simulink model "UPQC_model"  (R2020b)
settings: Solver=FixedStepAuto  StartTime=0.0  StopTime=Tsim  FixedStep=Tsample  MaxStep=Tsample  RelTol=1e-3
values from neighbouring files (symbols this model uses):
  C_parallel_Series = zeros(1,4)    [Netzmodell_Ini_DL.m]    (also in workspace_Ini.mat = [1e-05 1e-05 1e-05 0])
  C_parallel_Shunt = zeros(1,4)    [Netzmodell_Ini_DL.m]    (also in workspace_Ini.mat = [1e-05 1e-05 1e-05 0])
  CC_Ki = 5    [Netzmodell_Ini_DL.m]    (also in workspace_Ini.mat)
  CC_Ki_geg = 5    [Netzmodell_Ini_DL.m]    (also in workspace_Ini.mat)
  CC_Kp = 10    [Netzmodell_Ini_DL.m]    (also in workspace_Ini.mat)
  CC_Kp_geg = 10    [Netzmodell_Ini_DL.m]    (also in workspace_Ini.mat)
  CC_OS =     [workspace_Ini.mat]
  Czk = Szenario.Czk*u    [Netzmodell_Ini_DL.m]    (also in workspace_Ini.mat = 0.003)
  fak_RVC = Szenario.fak_RVC    [Netzmodell_Ini_DL.m]    (also in workspace_Ini.mat = [1 1 1])
  fak_Uns = [1; 1; 1]    [Netzmodell_Ini_DL.m]    (also in workspace_Ini.mat = [1 1 1])
  Flicker_Schaltzeitpunkte_L1 = Schaltzeitpunkte(1,:)    [Netzmodell_Ini_DL.m]    (also in workspace_Ini.mat = 10.5)
  Flicker_Schaltzeitpunkte_L2 = Schaltzeitpunkte(2,:)    [Netzmodell_Ini_DL.m]    (also in workspace_Ini.mat = 10.5)
  Flicker_Schaltzeitpunkte_L3 = Schaltzeitpunkte(3,:)    [Netzmodell_Ini_DL.m]    (also in workspace_Ini.mat = 10.5)
  fs = [f_nom; f_nom; f_nom]    [Netzmodell_Ini_DL.m]    (also in workspace_Ini.mat = [50 50 50])
  fsw = Szenario.fsw*k    [Netzmodell_Ini_DL.m]    (also in workspace_Ini.mat = 20000)
  I_Basis_Ober_L1 = I_Basis_Ober(1)    [Netzmodell_Ini_DL.m]    (also in workspace_Ini.mat = 0)
  I_Basis_Ober_L2 = I_Basis_Ober(2)    [Netzmodell_Ini_DL.m]    (also in workspace_Ini.mat = 0)
  I_Basis_Ober_L3 = I_Basis_Ober(3)    [Netzmodell_Ini_DL.m]    (also in workspace_Ini.mat = 0)
  I_relativ_Ober_L1 = Szenario.I_relativ_Ober_L1    [Netzmodell_Ini_DL.m]    (also in workspace_Ini.mat = [0 100 0 100 100 0 100 100 0 0 0 0 ... (50 elements, 1x50)])
  I_relativ_Ober_L2 = Szenario.I_relativ_Ober_L2    [Netzmodell_Ini_DL.m]    (also in workspace_Ini.mat = [0 100 0 100 100 0 100 100 0 0 0 0 ... (50 elements, 1x50)])
  I_relativ_Ober_L3 = Szenario.I_relativ_Ober_L3    [Netzmodell_Ini_DL.m]    (also in workspace_Ini.mat = [0 100 0 100 100 0 100 100 0 0 0 0 ... (50 elements, 1x50)])
  L_Ausgang_Series = zeros(1,4)    [Netzmodell_Ini_DL.m]    (also in workspace_Ini.mat = [0.00093 0.00093 0.00093 0.00093])
  L_Ausgang_Shunt = zeros(1,4)    [Netzmodell_Ini_DL.m]    (also in workspace_Ini.mat = [0.00093 0.00093 0.00093 0.00093])
  L_Eingang_Series = zeros(1,4)    [Netzmodell_Ini_DL.m]    (also in workspace_Ini.mat = [0.00085 0.00085 0.00085 0.00085])
  L_Eingang_Shunt = zeros(1,4)    [Netzmodell_Ini_DL.m]    (also in workspace_Ini.mat = [0.00085 0.00085 0.00085 0.00085])
  Ls_in = 52.2*u/10    (= 5.22e-06)    [Netzmodell_Ini_DL.m]    (also in workspace_Ini.mat)
  Ltrans = Szenario.Ltrans*m    [Netzmodell_Ini_DL.m]    (also in workspace_Ini.mat = 0.000256)
  OS_off = 6    [Netzmodell_Ini_DL.m]    (also in workspace_Ini.mat)
  OS_on = 1    [Netzmodell_Ini_DL.m]    (also in workspace_Ini.mat)
  Phi_Ober_L1 = Phi_Ober(1)    [Netzmodell_Ini_DL.m]    (also in workspace_Ini.mat = 0)
  Phi_Ober_L2 = Phi_Ober(2)    [Netzmodell_Ini_DL.m]    (also in workspace_Ini.mat = -120)
  Phi_Ober_L3 = Phi_Ober(3)    [Netzmodell_Ini_DL.m]    (also in workspace_Ini.mat = 120)
  Phis = [0; -120; 120]    [Netzmodell_Ini_DL.m]    (also in workspace_Ini.mat = [0 -120 120])
  Pl_Flicker = Pl_Flicker*k    [Netzmodell_Ini_DL.m]    (also in workspace_Ini.mat = [5000 5000 5000])
  Pl_Grund = Szenario.Pl_Grund *k    [Netzmodell_Ini_DL.m]    (also in workspace_Ini.mat = [5 5 5])
  Pl_RVC = Pl_RVC*k    [Netzmodell_Ini_DL.m]    (also in workspace_Ini.mat = [10000 10000 10000])
  Pl_Uns = Pl_Uns*k    [Netzmodell_Ini_DL.m]    (also in workspace_Ini.mat = [25000 10 10])
  Ql_ind_Flicker = Ql_ind_Flicker*k    [Netzmodell_Ini_DL.m]    (also in workspace_Ini.mat = [0 0 0])
  Ql_ind_Grund = Szenario.Ql_ind_Grund*k    [Netzmodell_Ini_DL.m]    (also in workspace_Ini.mat = [0 0 0])
  Ql_ind_RVC = Szenario.Ql_ind_RVC*k    [Netzmodell_Ini_DL.m]    (also in workspace_Ini.mat = [0 0 0])
  Ql_ind_Uns = Ql_ind_Uns*k    [Netzmodell_Ini_DL.m]    (also in workspace_Ini.mat = [0 0 0])
  Ql_kap_Flicker = Ql_kap_Flicker*k    [Netzmodell_Ini_DL.m]    (also in workspace_Ini.mat = [0 0 0])
  Ql_kap_Grund = Szenario.Ql_kap_Grund*k    [Netzmodell_Ini_DL.m]    (also in workspace_Ini.mat = [0 0 0])
  Ql_kap_RVC = Szenario.Ql_kap_RVC*k    [Netzmodell_Ini_DL.m]    (also in workspace_Ini.mat = [0 0 0])
  Ql_kap_Uns = Ql_kap_Uns*k    [Netzmodell_Ini_DL.m]    (also in workspace_Ini.mat = [0 0 0])
  R_Ausgang_Series = zeros(1,4)    [Netzmodell_Ini_DL.m]    (also in workspace_Ini.mat = [0.1 0.1 0.1 0.1])
  R_Ausgang_Shunt = zeros(1,4)    [Netzmodell_Ini_DL.m]    (also in workspace_Ini.mat = [0.1 0.1 0.1 0.1])
  R_Eingang_Series = zeros(1,4)    [Netzmodell_Ini_DL.m]    (also in workspace_Ini.mat = [0.1 0.1 0.1 0.1])
  R_Eingang_Shunt = zeros(1,4)    [Netzmodell_Ini_DL.m]    (also in workspace_Ini.mat = [0.1 0.1 0.1 0.1])
  R_parallel_Series = zeros(1,4)    [Netzmodell_Ini_DL.m]    (also in workspace_Ini.mat = [13 13 13 0])
  R_parallel_Shunt = zeros(1,4)    [Netzmodell_Ini_DL.m]    (also in workspace_Ini.mat = [13 13 13 0])
  R_ZK_Belastung = 20    [Netzmodell_Ini_DL.m]    (also in workspace_Ini.mat)
  Rs_in = 5.2*m/10    (= 0.00052)    [Netzmodell_Ini_DL.m]    (also in workspace_Ini.mat)
  Rtrans = Szenario.Rtrans    [Netzmodell_Ini_DL.m]    (also in workspace_Ini.mat = 0.206)
  RVC_L1_on_off_Zeitpunkte = Szenario.RVC_L1_on_off_Zeitpunkte    [Netzmodell_Ini_DL.m]    (also in workspace_Ini.mat = [10.5 40 10 11 12 13 14 15])
  RVC_L2_on_off_Zeitpunkte = Szenario.RVC_L2_on_off_Zeitpunkte    [Netzmodell_Ini_DL.m]    (also in workspace_Ini.mat = [10.5 40 10 11 12 13 14 15])
  RVC_L3_on_off_Zeitpunkte = Szenario.RVC_L3_on_off_Zeitpunkte    [Netzmodell_Ini_DL.m]    (also in workspace_Ini.mat = [10.5 40 10 11 12 13 14 15])
  RVC_off = 20.5    [Netzmodell_Ini_DL.m]    (also in workspace_Ini.mat)
  RVC_on = 20    [Netzmodell_Ini_DL.m]    (also in workspace_Ini.mat)
  RVC_val = [0.8,0.8,0.8]    [Netzmodell_Ini_DL.m]    (also in workspace_Ini.mat = [0.8 0.8 0.8])
  strans = Szenario.strans    [Netzmodell_Ini_DL.m]    (also in workspace_Ini.mat = 0.25)
  t_breaker_series = tacts    [Netzmodell_Ini_DL.m]    (also in workspace_Ini.mat = 0.5)
  tact = Szenario.tact    [Netzmodell_Ini_DL.m]    (also in workspace_Ini.mat = 0.5)
  tact_OS_Regler = Szenario.tact_OS_Regler    [Netzmodell_Ini_DL.m]    (also in workspace_Ini.mat = 0.5)
  tact_QU = 10    [Netzmodell_Ini_DL.m]    (also in workspace_Ini.mat)
  tacts = Szenario.tacts    [Netzmodell_Ini_DL.m]    (also in workspace_Ini.mat = 0.5)
  Tsample = Szenario.Tsample    [Netzmodell_Ini_DL.m]    (also in workspace_Ini.mat = 5e-06)
  Uns_L1_on_off_Zeitpunkte = Szenario.Uns_L1_on_off_Zeitpunkte    [Netzmodell_Ini_DL.m]    (also in workspace_Ini.mat = [1 6 10 11 12 13 14 15])
  Uns_L2_on_off_Zeitpunkte = Szenario.Uns_L2_on_off_Zeitpunkte    [Netzmodell_Ini_DL.m]    (also in workspace_Ini.mat = [10 30 10 11 12 13 14 15])
  Uns_L3_on_off_Zeitpunkte = Szenario.Uns_L3_on_off_Zeitpunkte    [Netzmodell_Ini_DL.m]    (also in workspace_Ini.mat = [10 30 10 11 12 13 14 15])
  Us = [Us_Amp; Us_Amp; Us_Amp]    [Netzmodell_Ini_DL.m]    (also in workspace_Ini.mat = [326.598632371 326.598632371 326.598632371])
  Us_Amp = sqrt(2)*400/sqrt(3)    [Netzmodell_Ini_DL.m]    (also in workspace_Ini.mat = 326.598632371)
  VC_Ki_gegen = 30    [Netzmodell_Ini_DL.m]    (also in workspace_Ini.mat)
  VC_Ki_gegen_shunt = 15    [Netzmodell_Ini_DL.m]    (also in workspace_Ini.mat)
  VC_Ki_mit = 5    [Netzmodell_Ini_DL.m]    (also in workspace_Ini.mat)
  VC_Kp_gegen = 5    [workspace_Ini.mat]
  VC_Kp_gegen_shunt = 2    [Netzmodell_Ini_DL.m]    (also in workspace_Ini.mat)
  VC_Kp_mit = 10    [Netzmodell_Ini_DL.m]    (also in workspace_Ini.mat)
  VC_ZK_Ki = 5    [Netzmodell_Ini_DL.m]    (also in workspace_Ini.mat)
  VC_ZK_Kp = 0.5    [Netzmodell_Ini_DL.m]    (also in workspace_Ini.mat)
  Vielfache_Ober_L1 = Szenario.Vielfache_Ober_L1    [Netzmodell_Ini_DL.m]    (also in workspace_Ini.mat = [1 2 3 4 5 6 7 8 9 10 11 12 ... (50 elements, 1x50)])
  Vielfache_Ober_L2 = Szenario.Vielfache_Ober_L2    [Netzmodell_Ini_DL.m]    (also in workspace_Ini.mat = [1 2 3 4 5 6 7 8 9 10 11 12 ... (50 elements, 1x50)])
  Vielfache_Ober_L3 = Szenario.Vielfache_Ober_L3    [Netzmodell_Ini_DL.m]    (also in workspace_Ini.mat = [1 2 3 4 5 6 7 8 9 10 11 12 ... (50 elements, 1x50)])
  ZK_Belastung_off = 100    [Netzmodell_Ini_DL.m]    (also in workspace_Ini.mat)
  ZK_Belastung_on = 100    [Netzmodell_Ini_DL.m]    (also in workspace_Ini.mat)
  Zwischenkreisspannung = 700    [Netzmodell_Ini_DL.m]    (also in workspace_Ini.mat)
undefined symbols (not defined in the file or in its folder): LAusgang, RReiheL3
libraries: powerlib x221, powerlib_meascontrol x80, pid_lib x23, eeTransforms x4, eePwmGeneratorTwoLevel x2, dspstat3 x1
(part 1 of 16)
settings Model: SimulationMode=accelerator  Creator=Emil Weymann  LastModifiedBy=gu92jek
settings SolverCC: ZeroCrossControl=DisableAll  ZeroCrossAlgorithm=Adaptive  AlgebraicLoopSolver=LineSearch
settings DataIOCC: SaveFormat=StructureWithTime  ReturnWorkspaceOutputs=off  LoggingFileName=Messdaten/RVC.mat
settings DebuggingCC: IgnoredZcDiagnostic=none

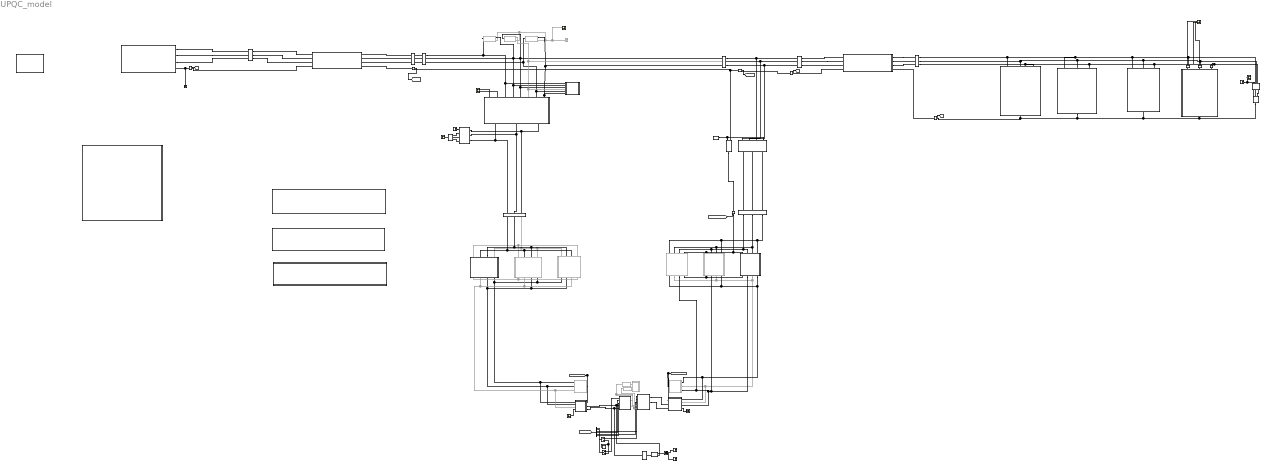
== system UPQC_model ==
  note: Zwischenkreis
  note: Wechselrichter Shunt
  note: Wechselrichter Series
  note: C
  note: (E) Messung Series UPQC
  note: Series Filter UPQC
  note: Shunt Filter UPQC
  note: (D) Messung Shunt UPQC
  note: ON / OFF Series UPQC
  note: (B) Messung UPQC
  note: (C) Messung Last
  note: (A) Messung Ortsnetzstation
  note: Power GUI Block
  note: Leitung
  note: Ortsnetzstation
  note: Lasten
  note: Grundlast
  note: Oberschwingungen Last
  note: Flicker Last
  note: Unsymmetrie Last
  note: RVC Last
  note: ON / OFF Shunt UPQC
  note: B
  note: E
  note: D
  note: A
  note: Messen
  note: Regelung UPQC
  note: Shunt
  note: Series
  note: PLL
  note: Leitung
  note: H
  note: G
  Add : Sum  Inputs=+-
  Breaker Series Control : Step  Commented=on  Time=t_breaker_series  Before=1  SampleTime=0
  Breaker Series Control1 : Step  Time=t_breaker_series  Before=1  After=0  SampleTime=0
  Breaker Shunt Control : powerlib_meascontrol/Pulse & Signal Generators/Stair Generator  t=t_breaker_shunt  e=1  Ts=0
  BreakerCtrlSig_Scope : Scope
  Bus Creator : BusCreator  Inputs=6
  Constant : Constant  Value=700
  Current Measurement{,1..4,6..9} (9 alike) : powerlib/Measurements/Current Measurement  PhasorSimulation=off  OutputType=Complex  PSBequivalent=0
  DC_Quelle_Zwischenkreis : Subsystem  Commented=on  mask{U_Zwischenkreis=Zwischenkreisspannung}
      mask prompts: U_Zwischenkreis "Zwischenkreisspannung [V]"
  Flicker Last : Subsystem  mask{wirk_L1=Pl_Flicker(1), blind_ind_L1=Ql_ind_Flicker(1), blind_kap_L1=Ql_kap_Flicker(1), Schaltzeitpunkte_L1=Flicker_Schaltzeitpunkte_L1, wirk_L2=Pl_Flicker(2), blind_ind_L2=Ql_ind_Flicker(2), blind_kap_L2=Ql_kap_Flicker(2), Schaltzeitpunkte_L2=Flicker_Schaltzeitpunkte_L2, wirk_L3=Pl_Flicker(3), blind_ind_L3=Ql_ind_Flicker(3), blind_kap_L3=Ql_kap_Flicker(3), Schaltzeitpunkte_L3=Flicker_Schaltzeitpunkte_L3}
      mask prompts: wirk_L1 "Wirkleistung[Watt]"; blind_ind_L1 "Blindleistung(Induktiv)[Var]"; blind_kap_L1 "Blindleistung(kapazitiv)[Var]"; Schaltzeitpunkte_L1 "Schaltzeitpunkte"; wirk_L2 "Wirkleistung[Watt]"; blind_ind_L2 "Blindleistung(Induktiv)[Var]"; blind_kap_L2 "Blindleistung(kapazitiv)[Var]"; Schaltzeitpunkte_L2 "Schaltzeitpunkte"; wirk_L3 "Wirkleistung[Watt]"; blind_ind_L3 "Blindleistung(Induktiv)[Var]"; blind_kap_L3 "Blindleistung(kapazitiv)[Var]"; Schaltzeitpunkte_L3 "Schaltzeitpunkte"
      mask DialogControl L1 Prompt: L1
      mask DialogControl L2 Prompt: L2
      mask DialogControl L3 Prompt: L3
  FreilaufDioden_Scope : Scope
  Freilaufdioden : Subsystem
  Ground2 : powerlib/Elements/Ground  LConnTagsString=a
  Grundlast : powerlib/Elements/Three-Phase Parallel RLC Load  LConnTagsString=A|B|C  RConnTagsString=N  Configuration=Y (neutral)  NominalVoltage=1000  Vabc=[400/sqrt(3) 400/sqrt(3) 400/sqrt(3)]  Vabcp=[1e3 1e3 1e3]  NominalFrequency=50  UnbalancedPower=on  ActivePower=10e3  InductivePower=100  CapacitivePower=100  Pabc=[Pl_Grund(1) Pl_Grund(2) Pl_Grund(3)]  QLabc=[Ql_ind_Grund(1) Ql_ind_Grund(2) Ql_ind_Grund(3)]  QCabc=[Ql_kap_Grund(1) Ql_kap_Grund(2) Ql_kap_Grund(3)]  Pabcp=[10e3 9e3 11e3]  QLabcp=[100 90 110]  QCabcp=[100 90 110]  Measurements=None  LoadType=constant PQ
  I_Last_Oberschwingung_Scope : Scope  NumInputPorts=3
  Ideal Switch : powerlib/Power Electronics/Ideal Switch  Ron=0.001  Lon=0  IC=0  Rs=inf  Cs=inf  Measurements=on
  L Filter Series : Subsystem  Commented=on  mask{LEinL1=L_Eingang_Series(1,1), REinL1=R_Eingang_Series(1,1), LEinL2=L_Eingang_Series(1,2), REinL2=R_Eingang_Series(1,2), LEinL3=L_Eingang_Series(1,3), REinL3=R_Eingang_Series(1,3), LEinN=L_Eingang_Series(1,4), REinN=R_Eingang_Series(1,4)}
      mask prompts: LEinL1 "L_Eingang[H]"; REinL1 "R_Eingang[Ohm]"; LEinL2 "L_Eingang[H]"; REinL2 "R_Eingang[Ohm]"; LEinL3 "L_Eingang[H]"; REinL3 "R_Eingang[Ohm]"; LEinN "L_Eingang[H]"; REinN "R_Eingang[Ohm]"
      mask DialogControl ParameterGroupVar Prompt: Parameter für den Filter
      mask DialogControl ContainerL1 Prompt: L1
      mask DialogControl ContainerL2 Prompt: L2
      mask DialogControl ContainerL3 Prompt: L3
      mask DialogControl ContainerN Prompt: N
  L Filter Shunt : Subsystem  Commented=on  mask{LEinL1=L_Eingang_Shunt(1,1), REinL1=R_Eingang_Shunt(1,1), LEinL2=L_Eingang_Shunt(1,2), REinL2=R_Eingang_Shunt(1,2), LEinL3=L_Eingang_Shunt(1,3), REinL3=R_Eingang_Shunt(1,3), LEinN=L_Eingang_Shunt(1,4), REinN=L_Eingang_Shunt(1,4)}
      mask prompts: LEinL1 "L_Eingang[H]"; REinL1 "R_Eingang[Ohm]"; LEinL2 "L_Eingang[H]"; REinL2 "R_Eingang[Ohm]"; LEinL3 "L_Eingang[H]"; REinL3 "R_Eingang[Ohm]"; LEinN "L_Eingang[H]"; REinN "R_Eingang[Ohm]"
      mask DialogControl ParameterGroupVar Prompt: Parameter für den Filter
      mask DialogControl ContainerL1 Prompt: L1
      mask DialogControl ContainerL2 Prompt: L2
      mask DialogControl ContainerL3 Prompt: L3
      mask DialogControl ContainerN Prompt: N
  L1 Breaker Series : powerlib/Elements/Breaker  Commented=on  InitialState=1  SwitchingTimes="[1/60  5/60]"  External=on  BreakerResistance=0.01  SnubberResistance=1e6  SnubberCapacitance=inf  Measurements=None  MoreParameters=on  NoBreakLoop=off
  L2 Breaker Series : powerlib/Elements/Breaker  Commented=on  InitialState=1  SwitchingTimes="[1/60  5/60]"  External=on  BreakerResistance=0.01  SnubberResistance=1e6  SnubberCapacitance=inf  Measurements=None  MoreParameters=on  NoBreakLoop=off
  L3 Breaker Series : powerlib/Elements/Breaker  Commented=on  InitialState=1  SwitchingTimes="[1/60  5/60]"  External=on  BreakerResistance=0.01  SnubberResistance=1e6  SnubberCapacitance=inf  Measurements=None  MoreParameters=on  NoBreakLoop=off
  LC Filter Series : Subsystem  Commented=on  mask{LEinL1=L_Eingang_Series(1,1)*3, CL1=C_parallel_Series(1,1)*750, REinL1=R_Eingang_Series(1,1), RReiheL1=R_parallel_Series(1,1), LEinL2=L_Eingang_Series(1,2)*3, CL2=C_parallel_Series(1,2)*750, REinL2=R_Eingang_Series(1,2), RReiheL2=R_parallel_Series(1,2), LEinL3=L_Eingang_Series(1,3)*3, CL3=C_parallel_Series(1,3)*750, REinL3=R_Eingang_Series(1,3), RReiheL3=R_parallel_Series(1,3), LEinN=L_Eingang_Series(1,4), REinN=R_Eingang_Series(1,4)}
      mask prompts: LEinL1 "L_Eingang[H]"; CL1 "C[F]"; REinL1 "R_Eingang[Ohm]"; RReiheL1 "R in Reihe C[Ohm]"; LEinL2 "L_Eingang[H]"; CL2 "C[F]"; REinL2 "R_Eingang[Ohm]"; RReiheL2 "R in Reihe C[Ohm]"; LEinL3 "L_Eingang[H]"; CL3 "C[F]"; REinL3 "R_Eingang[Ohm]"; RReiheL3 "R in Reihe C[Ohm]"; LEinN "L_Eingang[H]"; REinN "R_Eingang[Ohm]"
      mask DialogControl ParameterGroupVar Prompt: Parameter für den Filter
      mask DialogControl ContainerL1 Prompt: L1
      mask DialogControl ContainerL2 Prompt: L2
      mask DialogControl ContainerL3 Prompt: L3
      mask DialogControl ContainerN Prompt: N
  LC Filter Shunt : Subsystem  Commented=on  mask{LEinL1=L_Eingang_Shunt(1,1), CL1=C_parallel_Shunt(1,1), REinL1=R_Eingang_Shunt(1,1), RReiheL1=R_parallel_Shunt(1,1), LEinL2=L_Eingang_Shunt(1,2), CL2=C_parallel_Shunt(1,2), REinL2=R_Eingang_Shunt(1,2), RReiheL2=R_parallel_Shunt(1,2), LEinL3=L_Eingang_Shunt(1,3), CL3=C_parallel_Shunt(1,3), REinL3=R_Eingang_Shunt(1,3), RReiheL3=R_parallel_Shunt(1,3), LEinN=0, REinN=0}
      mask prompts: LEinL1 "L_Eingang[H]"; CL1 "C[F]"; REinL1 "R_Eingang[Ohm]"; RReiheL1 "R in Reihe C[Ohm]"; LEinL2 "L_Eingang[H]"; CL2 "C[F]"; REinL2 "R_Eingang[Ohm]"; RReiheL2 "R in Reihe C[Ohm]"; LEinL3 "L_Eingang[H]"; CL3 "C[F]"; REinL3 "R_Eingang[Ohm]"; RReiheL3 "R in Reihe C[Ohm]"; LEinN "L_Eingang[H]"; REinN "R_Eingang[Ohm]"
      mask DialogControl ParameterGroupVar Prompt: Parameter für den Filter
      mask DialogControl ContainerL1 Prompt: L1
      mask DialogControl ContainerL2 Prompt: L2
      mask DialogControl ContainerL3 Prompt: L3
      mask DialogControl ContainerN Prompt: N
  LCL Filter Series : Subsystem  mask{LEinL1=L_Eingang_Series(1,1), LAusL1=L_Ausgang_Series(1,1), CL1=C_parallel_Series(1,1), REinL1=R_Eingang_Series(1,1), RAusL1=R_Ausgang_Series(1,1), RReiheL1=R_parallel_Series(1,1), LEinL2=L_Eingang_Series(1,2), LAusL2=L_Ausgang_Series(1,2), CL2=C_parallel_Series(1,2), REinL2=R_Eingang_Series(1,2), RAusL2=R_Ausgang_Series(1,2), RReiheL2=R_parallel_Series(1,2), LEinL3=L_Eingang_Series(1,3), LAusL3=L_Ausgang_Series(1,3), CL3=C_parallel_Series(1,3), REinL3=R_Eingang_Series(1,3), RAusL3=R_Ausgang_Series(1,3), RReiheL3=R_parallel_Series(1,3), LEinN=L_Eingang_Series(1,4), LAusN=L_Ausgang_Series(1,4), REinN=R_Eingang_Series(1,4), RAusN=R_Ausgang_Series(1,4)}
      mask prompts: LEinL1 "L_Eingang[H]"; LAusL1 "L_Ausgang[H]"; CL1 "C[F]"; REinL1 "R_Eingang[Ohm]"; RAusL1 "R_Ausgang[Ohm]"; RReiheL1 "R in Reihe C[Ohm]"; LEinL2 "L_Eingang[H]"; LAusL2 "L_Ausgang[H]"; CL2 "C[F]"; REinL2 "R_Eingang[Ohm]"; RAusL2 "R_Ausgang[Ohm]"; RReiheL2 "R in Reihe C[Ohm]"; LEinL3 "L_Eingang[H]"; LAusL3 "L_Ausgang[H]"; CL3 "C[F]"; REinL3 "R_Eingang[Ohm]"; RAusL3 "R_Ausgang[Ohm]"; RReiheL3 "R in Reihe C[Ohm]"; LEinN "L_Eingang[H]"; LAusN "L_Ausgang[H]"; REinN "R_Eingang[Ohm]"; RAusN "R_Ausgang[Ohm]"
      mask DialogControl ParameterGroupVar Prompt: Parameter für den Filter
      mask DialogControl ContainerL1 Prompt: L1
      mask DialogControl ContainerL2 Prompt: L2
      mask DialogControl ContainerL3 Prompt: L3
      mask DialogControl ContainerN Prompt: N
  LCL Filter Shunt : Subsystem  mask{LEinL1=L_Eingang_Shunt(1,1), LAusL1=L_Ausgang_Shunt(1,1), CL1=C_parallel_Shunt(1,1), REinL1=R_Eingang_Shunt(1,1), RAusL1=R_Ausgang_Shunt(1,1), RReiheL1=R_parallel_Shunt(1,1), LEinL2=L_Eingang_Shunt(1,2), LAusL2=L_Ausgang_Shunt(1,2), CL2=C_parallel_Shunt(1,2), REinL2=R_Eingang_Shunt(1,2), RAusL2=R_Ausgang_Shunt(1,2), RReiheL2=R_parallel_Shunt(1,2), LEinL3=L_Eingang_Shunt(1,3), LAusL3=L_Ausgang_Shunt(1,3), CL3=C_parallel_Shunt(1,3), REinL3=R_Eingang_Shunt(1,3), RAusL3=R_Ausgang_Shunt(1,3), RReiheL3=R_parallel_Shunt(1,3), LEinN=L_Eingang_Shunt(1,4), LAusN=L_Ausgang_Shunt(1,4), REinN=R_Eingang_Shunt(1,4), RAusN=R_Ausgang_Shunt(1,4)}
      mask prompts: LEinL1 "L_Eingang[H]"; LAusL1 "L_Ausgang[H]"; CL1 "C[F]"; REinL1 "R_Eingang[Ohm]"; RAusL1 "R_Ausgang[Ohm]"; RReiheL1 "R in Reihe C[Ohm]"; LEinL2 "L_Eingang[H]"; LAusL2 "L_Ausgang[H]"; CL2 "C[F]"; REinL2 "R_Eingang[Ohm]"; RAusL2 "R_Ausgang[Ohm]"; RReiheL2 "R in Reihe C[Ohm]"; LEinL3 "L_Eingang[H]"; LAusL3 "L_Ausgang[H]"; CL3 "C[F]"; REinL3 "R_Eingang[Ohm]"; RAusL3 "R_Ausgang[Ohm]"; RReiheL3 "R in Reihe C[Ohm]"; LEinN "L_Eingang[H]"; LAusN "L_Ausgang[H]"; REinN "R_Eingang[Ohm]"; RAusN "R_Ausgang[Ohm]"
      mask DialogControl ParameterGroupVar Prompt: Parameter für den Filter
      mask DialogControl ContainerL1 Prompt: L1
      mask DialogControl ContainerL2 Prompt: L2
      mask DialogControl ContainerL3 Prompt: L3
      mask DialogControl ContainerN Prompt: N
  Leitungsnachbildung RL : Subsystem  mask{R_pro_KM=Rtrans, L_pro_KM=Ltrans, KM=strans}
      mask prompts: R_pro_KM "Widerstandsbelag(Ohm_pro_KM)"; L_pro_KM "Induktivitätsbelag(H_pro_KM)"; KM "Länge(Km)"
  Leitungsnachbildung RL1 : Subsystem  mask{R_pro_KM=Rtrans, L_pro_KM=Ltrans, KM=strans}
      mask prompts: R_pro_KM "Widerstandsbelag(Ohm_pro_KM)"; L_pro_KM "Induktivitätsbelag(H_pro_KM)"; KM "Länge(Km)"
  Manual Switch : ManualSwitch
  Manual Switch1 : ManualSwitch
  Measurement Transformer : Subsystem
  Messpunkt C : powerlib/Measurements/Three-Phase V-I Measurement  VoltageMeasurement=phase-to-ground  SetLabelV=on  LabelV=Vabc_C  Vpu=off  VpuLL=off  CurrentMeasurement=yes  SetLabelI=on  LabelI=Iabc_C  Ipu=off  Pbase=100e6  Vbase=500e3  OutputType=Complex  PhasorSimulation=off  PSBequivalent=0
  Messpunkt G : powerlib/Measurements/Three-Phase V-I Measurement  VoltageMeasurement=phase-to-ground  SetLabelV=on  LabelV=Vabc_G  Vpu=off  VpuLL=off  CurrentMeasurement=yes  SetLabelI=on  LabelI=Iabc_G  Ipu=off  Pbase=100e6  Vbase=500e3  OutputType=Complex  PhasorSimulation=off  PSBequivalent=0
  Messpunkt H : powerlib/Measurements/Three-Phase V-I Measurement  VoltageMeasurement=phase-to-ground  SetLabelV=on  LabelV=Vabc_H  Vpu=off  VpuLL=off  CurrentMeasurement=yes  SetLabelI=on  LabelI=Iabc_H  Ipu=off  Pbase=100e6  Vbase=500e3  OutputType=Complex  PhasorSimulation=off  PSBequivalent=0
  Messsignale : Subsystem
  N Breaker Shunt : powerlib/Elements/Breaker  InitialState=0  SwitchingTimes="[1/60  5/60]"  External=on  BreakerResistance=0.01  SnubberResistance=1e6  SnubberCapacitance=inf  Measurements=None  MoreParameters=on  NoBreakLoop=off
  Oberschwingung Last : Subsystem  mask{amp_L1=I_relativ_Ober_L1, BasisStromL1=I_Basis_Ober_L1, O_L1=Vielfache_Ober_L1, phase_L1=Phi_Ober_L1, init_amp_L1=0, init_phase_L1=0, init_freq_L1=50, amp_L2=I_relativ_Ober_L2, BasisStromL2=I_Basis_Ober_L2, O_L2=Vielfache_Ober_L2, phase_L2=Phi_Ober_L2, init_amp_L2=0, init_phase_L2=0, init_freq_L2=50, amp_L3=I_relativ_Ober_L3, BasisStromL3=I_Basis_Ober_L3, O_L3=Vielfache_Ober_L3, phase_L3=Phi_Ober_L3, init_amp_L3=0, init_phase_L3=0, init_freq_L3=50}
      mask prompts: amp_L1 "Amplitude von Basistrom(50Hz)[%] (Dimension n)"; BasisStromL1 "Basisstrom (bei 50Hz oder 1.Harmonische) [A] (Dimension 1)"; O_L1 "Vielfache von 50 Hz (Dimension n)"; phase_L1 "Phase[Grad] (Dimension 1)"; init_amp_L1 "Initial_Amplitude[A] (Dimension 1)"; init_phase_L1 "Initial_Phase[Grad] (Dimension 1)"; init_freq_L1 "Initial_Frequenz[Hz] (Dimension 1)"; amp_L2 "Amplitude von Basistrom(50Hz)[%] (Dimension n)"; BasisStromL2 "Basisstrom (bei 50Hz oder 1.Harmonische) [A] (Dimension 1)"; O_L2 "Vielfache von 50 Hz (Dimension n)"; phase_L2 "Phase[Grad] (Dimension 1)"; init_amp_L2 "Initial_Amplitude[A] (Dimension 1)"; init_phase_L2 "Initial_Phase[Grad] (Dimension 1)"; init_freq_L2 "Initial_Frequenz[Hz] (Dimension 1)"; amp_L3 "Amplitude von Basistrom(50Hz)[%] (Dimension n)"; BasisStromL3 "Basisstrom (bei 50Hz oder 1.Harmonische) [A] (Dimension 1)"; O_L3 "Vielfache von 50 Hz (Dimension n)"; phase_L3 "Phase[Grad] (Dimension 1)"; init_amp_L3 "Initial_Amplitude[A] (Dimension 1)"; init_phase_L3 "Initial_Phase[Grad] (Dimension 1)"; init_freq_L3 "Initial_Frequenz[Hz] (Dimension 1)"
      mask DialogControl L1 Prompt: L1
      mask DialogControl L2 Prompt: L2
      mask DialogControl L3 Prompt: L3
  Position 1 : powerlib/Measurements/Three-Phase V-I Measurement  VoltageMeasurement=phase-to-ground  SetLabelV=on  LabelV=Vabc_A  Vpu=off  VpuLL=off  CurrentMeasurement=yes  SetLabelI=on  LabelI=Iabc_A  Ipu=off  Pbase=100e6  Vbase=500e3  OutputType=Complex  PhasorSimulation=off  PSBequivalent=0
  Position 2 : powerlib/Measurements/Three-Phase V-I Measurement  VoltageMeasurement=phase-to-ground  SetLabelV=on  LabelV=Vabc_B  Vpu=off  VpuLL=off  CurrentMeasurement=yes  SetLabelI=on  LabelI=Iabc_B  Ipu=off  Pbase=100e6  Vbase=500e3  OutputType=Complex  PhasorSimulation=off  PSBequivalent=0
  Position 3 : powerlib/Measurements/Three-Phase V-I Measurement  VoltageMeasurement=phase-to-phase  SetLabelV=on  LabelV=Vabc_B_pp  Vpu=off  VpuLL=off  CurrentMeasurement=no  SetLabelI=on  LabelI=Iabc_B  Ipu=off  Pbase=100e6  Vbase=500e3  OutputType=Complex  PhasorSimulation=off  PSBequivalent=0
  RVC Last : Subsystem  mask{wirk_L1=Pl_RVC(1), blind_ind_L1=Ql_ind_RVC(1), blind_kap_L1=Ql_kap_RVC(1), faktor_L1=fak_RVC(1), t1_L1=RVC_L1_on_off_Zeitpunkte(1), t1_L1_off=RVC_L1_on_off_Zeitpunkte(2), t2_L1=RVC_L1_on_off_Zeitpunkte(3), t2_L1_off=RVC_L1_on_off_Zeitpunkte(4), t3_L1=RVC_L1_on_off_Zeitpunkte(5), t3_L1_off=RVC_L1_on_off_Zeitpunkte(6), t4_L1=RVC_L1_on_off_Zeitpunkte(7), t4_L1_off=RVC_L1_on_off_Zeitpunkte(8), wirk_L2=Pl_RVC(2), blind_ind_L2=Ql_ind_RVC(2), blind_kap_L2=Ql_kap_RVC(2), faktor_L2=fak_RVC(2), t1_L2=RVC_L2_on_off_Zeitpunkte(1), t1_L2_off=RVC_L2_on_off_Zeitpunkte(2), t2_L2=RVC_L2_on_off_Zeitpunkte(3), t2_L2_off=RVC_L2_on_off_Zeitpunkte(4), t3_L2=RVC_L2_on_off_Zeitpunkte(5), t3_L2_off=RVC_L2_on_off_Zeitpunkte(6), t4_L2=RVC_L2_on_off_Zeitpunkte(7), t4_L2_off=RVC_L2_on_off_Zeitpunkte(8), wirk_L3=Pl_RVC(3), blind_ind_L3=Ql_ind_RVC(3), blind_kap_L3=Ql_kap_RVC(3), faktor_L3=fak_RVC(3), t1_L3=RVC_L3_on_off_Zeitpunkte(1), t1_L3_off=RVC_L3_on_off_Zeitpunkte(2), t2_L3=RVC_L3_on_off_Zeitpunkte(3), t2_L3_off=RVC_L3_on_off_Zeitpunkte(4), t3_L3=RVC_L3_on_off_Zeitpunkte(5), t3_L3_off=RVC_L3_on_off_Zeitpunkte(6), t4_L3=RVC_L3_on_off_Zeitpunkte(7), t4_L3_off=RVC_L3_on_off_Zeitpunkte(8)}
      mask prompts: wirk_L1 "Wirkleistung[Watt]"; blind_ind_L1 "Blindleistung(Induktiv)[Var]"; blind_kap_L1 "Blindleistung(kapazitiv)[Var]"; faktor_L1 "Faktor für Anstieg [2 = doppelt]"; t1_L1 "t1_on"; t1_L1_off "t1_off"; t2_L1 "t2_on"; t2_L1_off "t2_off"; t3_L1 "t3_on"; t3_L1_off "t3_off"; t4_L1 "t4_on"; t4_L1_off "t4_off"; wirk_L2 "Wirkleistung[Watt]"; blind_ind_L2 "Blindleistung(Induktiv)[Var]"; blind_kap_L2 "Blindleistung(kapazitiv)[Var]"; faktor_L2 "Faktor für Anstieg [2 = doppelt]"; t1_L2 "t1_on"; t1_L2_off "t1_off"; t2_L2 "t2_on"; t2_L2_off "t2_off"; t3_L2 "t3_on"; t3_L2_off "t3_off"; t4_L2 "t4_on"; t4_L2_off "t4_off"; wirk_L3 "Wirkleistung[Watt]"; blind_ind_L3 "Blindleistung(Induktiv)[Var]"; blind_kap_L3 "Blindleistung(kapazitiv)[Var]"; faktor_L3 "Faktor für Anstieg [2 = doppelt]"; t1_L3 "t1_on"; t1_L3_off "t1_off"; t2_L3 "t2_on"; t2_L3_off "t2_off"; t3_L3 "t3_on"; t3_L3_off "t3_off"; t4_L3 "t4_on"; t4_L3_off "t4_off"
      mask DialogControl L1 Prompt: L1
      mask DialogControl L2 Prompt: L2
      mask DialogControl L3 Prompt: L3
  Series RLC Branch1 : powerlib/Elements/Series RLC Branch  Commented=on  LConnTagsString=__new0  RConnTagsString=__new0  BranchType=R  Resistance=0.1  Inductance=1e-3  SetiL0=off  InitialCurrent=0  Capacitance=1e-6  Setx0=off  InitialVoltage=0  Measurements=None
  Series RLC Branch3 : powerlib/Elements/Series RLC Branch  Commented=on  LConnTagsString=__new0  RConnTagsString=__new0  BranchType=R  Resistance=0.1  Inductance=1e-3  SetiL0=off  InitialCurrent=0  Capacitance=1e-6  Setx0=off  InitialVoltage=0  Measurements=None
  Series RLC Branch4 : powerlib/Elements/Series RLC Branch  LConnTagsString=__new0  RConnTagsString=__new0  BranchType=R  Resistance=R_ZK_Belastung  Inductance=1e-3  SetiL0=off  InitialCurrent=0  Capacitance=1e-6  Setx0=off  InitialVoltage=0  Measurements=None
  Series UPQC : Subsystem
  Series UPQC1 : Subsystem
  Shunt Strom/ Spannung : powerlib/Measurements/Three-Phase V-I Measurement  VoltageMeasurement=phase-to-ground  SetLabelV=on  LabelV=Vabc_D  Vpu=off  VpuLL=off  CurrentMeasurement=yes  SetLabelI=on  LabelI=Iabc_D  Ipu=off  Pbase=100e6  Vbase=500e3  OutputType=Complex  PhasorSimulation=off  PSBequivalent=0
  Shunt UPQC : Subsystem
  Sollwertquelle_Series_U : Subsystem  Commented=on
  Sollwertquelle_Shunt_U : Subsystem  Commented=on
  Strom Spannung Trafowicklungen Primär : Scope  NumInputPorts=2
  Subsystem : Subsystem  mask{Amp_L1=Us(1), phase_L1=Phis(1), f_L1=fs(1), Amp_L2=Us(2), phase_L2=Phis(2), f_L2=fs(2), Amp_L3=Us(3), phase_L3=Phis(3), f_L3=fs(3), R=Rs_in, L=Ls_in}
      mask prompts: Amp_L1 "Amplitude_L1[V]"; phase_L1 "Phase_L1[Grad]"; f_L1 "Frequenz_L1[Hz]"; Amp_L2 "Amplitude_L2[V]"; phase_L2 "Phase_L2[Grad]"; f_L2 "Frequenz_L2[Hz]"; Amp_L3 "Amplitude_L3[V]"; phase_L3 "Phase_L3[Grad]"; f_L3 "Frequenz_L3[Hz]"
      mask DialogControl L1 Prompt: L1
      mask DialogControl L2 Prompt: L2
      mask DialogControl L3 Prompt: L3
      mask DialogControl Innenwiderstand Prompt: Spannungsquelle Innenwiderstand
  Switch_Grundlast_Scope : Scope
  Three-Phase Breaker : powerlib/Elements/Three-Phase Breaker  InitialState=closed  SwitchA=on  SwitchB=on  SwitchC=on  SwitchTimes="[1/60  5/60]"  External=on  BreakerResistance=0.01  SnubberResistance=1e6  SnubberCapacitance=inf  Measurements=None
  Three-Phase Breaker Shunt : powerlib/Elements/Three-Phase Breaker  InitialState=open  SwitchA=on  SwitchB=on  SwitchC=on  SwitchTimes="[1/60  5/60]"  External=on  BreakerResistance=0.01  SnubberResistance=1e6  SnubberCapacitance=inf  Measurements=None
  Three-Phase Breaker Shunt1 : powerlib/Elements/Three-Phase Breaker  InitialState=closed  SwitchA=on  SwitchB=on  SwitchC=on  SwitchTimes=[5000]  External=on  BreakerResistance=0.0001  SnubberResistance=100000  SnubberCapacitance=inf  Measurements=None
  Transformator mit Messung : Subsystem
      settings: PortSchema="{\"entries\":[{\"content\":{\"sides\":[{\"content\":{\"connectorIds\":[\"LConn1\",\"LConn2\",\"LConn3\"]},\"type\":\"ConnectorPlacement.EquallySpacedRectSide\",\"uuid\":\"1e79c22a-2718-4fc0-b2f9-9b892a96ea34\"},{\"content\":{\"connectorIds\":[\"RConn1\",\"RConn2\",\"RConn3\",\"RConn4\",\"RConn5\",\"RConn6\",\"Out1\",\"Out2\"],\"side\":\"RIGHT\"},\"type\":\"ConnectorPlacement.EquallySpacedRectSide\",\"uuid\":\"2c156bee-5cd3-4d63-88ab-2b5527aeb6f0\"},{\"content\":{\"connectorIds\":[],\"side\":\"TOP\"},\"type\":\"ConnectorPlacement.EquallySpacedRectSide\",\"uuid\":\"9e01bd14-a20e-4e29-ab52-7705115dd82d\"},{\"content\":{\"connectorIds\":[],\"side\":\"HIDDEN\"},\"type\":\"ConnectorPlacement.EquallySpacedRectSide\",\"uuid\":\"6f305824-b768-40e1-89ea-9ec84b042939\"}]},\"type\":\"ConnectorPlacement.EquallySpacedConnector\",\"uuid\":\"381d622f-826c-4b1a-a5e2-e3afd6f4e142\"}],\"packageUris\":[\"http://schema.mathworks.com/mf0/Connector/R2020b\"],\"version\":\"1.0\"}"
  Unsymmetrie Last : Subsystem  mask{wirk_L1=Pl_Uns(1), blind_ind_L1=Ql_ind_Uns(1), blind_kap_L1=Ql_kap_Uns(1), faktor_L1=fak_Uns(1), t1_L1=Uns_L1_on_off_Zeitpunkte(1), t1_L1_off=Uns_L1_on_off_Zeitpunkte(2), t2_L1=Uns_L1_on_off_Zeitpunkte(3), t2_L1_off=Uns_L1_on_off_Zeitpunkte(4), t3_L1=Uns_L1_on_off_Zeitpunkte(5), t3_L1_off=Uns_L1_on_off_Zeitpunkte(6), t4_L1=Uns_L1_on_off_Zeitpunkte(7), t4_L1_off=Uns_L1_on_off_Zeitpunkte(8), wirk_L2=Pl_Uns(2), blind_ind_L2=Ql_ind_Uns(2), blind_kap_L2=Ql_kap_Uns(2), faktor_L2=fak_Uns(2), t1_L2=Uns_L2_on_off_Zeitpunkte(1), t1_L2_off=Uns_L2_on_off_Zeitpunkte(2), t2_L2=Uns_L2_on_off_Zeitpunkte(3), t2_L2_off=Uns_L2_on_off_Zeitpunkte(4), t3_L2=Uns_L2_on_off_Zeitpunkte(5), t3_L2_off=Uns_L2_on_off_Zeitpunkte(6), t4_L2=Uns_L2_on_off_Zeitpunkte(7), t4_L2_off=Uns_L2_on_off_Zeitpunkte(8), wirk_L3=Pl_Uns(3), blind_ind_L3=Ql_ind_Uns(3), blind_kap_L3=Ql_kap_Uns(3), faktor_L3=fak_Uns(3), t1_L3=Uns_L3_on_off_Zeitpunkte(1), t1_L3_off=Uns_L3_on_off_Zeitpunkte(2), t2_L3=Uns_L3_on_off_Zeitpunkte(3), t2_L3_off=Uns_L3_on_off_Zeitpunkte(4), t3_L3=Uns_L3_on_off_Zeitpunkte(5), t3_L3_off=Uns_L3_on_off_Zeitpunkte(6), t4_L3=Uns_L3_on_off_Zeitpunkte(7), t4_L3_off=Uns_L3_on_off_Zeitpunkte(8)}
      mask prompts: wirk_L1 "Wirkleistung[Watt]"; blind_ind_L1 "Blindleistung(Induktiv)[Var]"; blind_kap_L1 "Blindleistung(kapazitiv)[Var]"; faktor_L1 "Faktor für Anstieg [2 = doppelt]"; t1_L1 "t1_on"; t1_L1_off "t1_off"; t2_L1 "t2_on"; t2_L1_off "t2_off"; t3_L1 "t3_on"; t3_L1_off "t3_off"; t4_L1 "t4_on"; t4_L1_off "t4_off"; wirk_L2 "Wirkleistung[Watt]"; blind_ind_L2 "Blindleistung(Induktiv)[Var]"; blind_kap_L2 "Blindleistung(kapazitiv)[Var]"; faktor_L2 "Faktor für Anstieg [2 = doppelt]"; t1_L2 "t1_on"; t1_L2_off "t1_off"; t2_L2 "t2_on"; t2_L2_off "t2_off"; t3_L2 "t3_on"; t3_L2_off "t3_off"; t4_L2 "t4_on"; t4_L2_off "t4_off"; wirk_L3 "Wirkleistung[Watt]"; blind_ind_L3 "Blindleistung(Induktiv)[Var]"; blind_kap_L3 "Blindleistung(kapazitiv)[Var]"; faktor_L3 "Faktor für Anstieg [2 = doppelt]"; t1_L3 "t1_on"; t1_L3_off "t1_off"; t2_L3 "t2_on"; t2_L3_off "t2_off"; t3_L3 "t3_on"; t3_L3_off "t3_off"; t4_L3 "t4_on"; t4_L3_off "t4_off"
      mask DialogControl L1 Prompt: L1
      mask DialogControl L2 Prompt: L2
      mask DialogControl L3 Prompt: L3
  VSC_Series_SPWM_Scope : Scope
  VSC_Series_U : Subsystem  mask{vdc=Zwischenkreisspannung, WR_takt=fsw}
      mask prompts: vdc "Zwischenkreisspannung"; WR_takt "Taktfrequenz Bruecken"
      settings: PortSchema="{\"entries\":[{\"content\":{\"sides\":[{\"content\":{\"connectorIds\":[\"In1\",\"LConn1\",\"LConn2\"]},\"type\":\"ConnectorPlacement.EquallySpacedRectSide\",\"uuid\":\"3324cbaa-554a-49d8-9410-bfd63029b390\"},{\"content\":{\"connectorIds\":[\"RConn1\",\"RConn2\",\"RConn3\",\"Out1\"],\"side\":\"RIGHT\"},\"type\":\"ConnectorPlacement.EquallySpacedRectSide\",\"uuid\":\"248b0aca-34b4-4104-9288-613037293863\"},{\"content\":{\"connectorIds\":[],\"side\":\"TOP\"},\"type\":\"ConnectorPlacement.EquallySpacedRectSide\",\"uuid\":\"fa218b61-03df-498c-bf3d-1318c3fff998\"},{\"content\":{\"connectorIds\":[],\"side\":\"HIDDEN\"},\"type\":\"ConnectorPlacement.EquallySpacedRectSide\",\"uuid\":\"0aa4873c-6f4a-4cae-b332-9f04d6bbd78c\"}]},\"type\":\"ConnectorPlacement.EquallySpacedConnector\",\"uuid\":\"aa15b3bc-645b-4460-89b4-99e6ebf003ce\"}],\"packageUris\":[\"http://schema.mathworks.com/mf0/Connector/R2020b\"],\"version\":\"1.0\"}"
  VSC_Shunt_SPWM_Scope : Scope
  VSC_Shunt_U : Subsystem  mask{vdc=Zwischenkreisspannung, WR_takt=fsw}
      mask prompts: vdc "Zwischenkreisspannung"; WR_takt "Taktfrequenz Bruecken"
      settings: PortSchema="{\"entries\":[{\"content\":{\"sides\":[{\"content\":{\"connectorIds\":[\"In1\",\"LConn1\",\"LConn2\"]},\"type\":\"ConnectorPlacement.EquallySpacedRectSide\",\"uuid\":\"3324cbaa-554a-49d8-9410-bfd63029b390\"},{\"content\":{\"connectorIds\":[\"RConn1\",\"RConn2\",\"RConn3\",\"Out1\"],\"side\":\"RIGHT\"},\"type\":\"ConnectorPlacement.EquallySpacedRectSide\",\"uuid\":\"248b0aca-34b4-4104-9288-613037293863\"},{\"content\":{\"connectorIds\":[],\"side\":\"TOP\"},\"type\":\"ConnectorPlacement.EquallySpacedRectSide\",\"uuid\":\"fa218b61-03df-498c-bf3d-1318c3fff998\"},{\"content\":{\"connectorIds\":[],\"side\":\"HIDDEN\"},\"type\":\"ConnectorPlacement.EquallySpacedRectSide\",\"uuid\":\"0aa4873c-6f4a-4cae-b332-9f04d6bbd78c\"}]},\"type\":\"ConnectorPlacement.EquallySpacedConnector\",\"uuid\":\"aa15b3bc-645b-4460-89b4-99e6ebf003ce\"}],\"packageUris\":[\"http://schema.mathworks.com/mf0/Connector/R2020b\"],\"version\":\"1.0\"}"
  Wechselrichter Reihe Strom/ Spannung : powerlib/Measurements/Three-Phase V-I Measurement  VoltageMeasurement=phase-to-ground  SetLabelV=on  LabelV=Vabc_E  Vpu=off  VpuLL=off  CurrentMeasurement=yes  SetLabelI=on  LabelI=Iabc_E  Ipu=off  Pbase=100e6  Vbase=500e3  OutputType=Complex  PhasorSimulation=off  PSBequivalent=0
  Zwischenkreis_Series : Subsystem  mask{C_Zwischenkreis=Czk}
      mask prompts: C_Zwischenkreis "Zwischenkreiskapazität [F]"
  Zwischenkreis_Shunt : Subsystem  mask{C_Zwischenkreis=Czk}
      mask prompts: C_Zwischenkreis "Zwischenkreiskapazität [F]"
  powergui : powerlib/powergui  Priority=1  SimulationMode=Discrete  SampleTime=Tsample  frequency=50  Iterations=50  frequencyindice=0  Pbase=100e6  ErrMax=1e-4  UnitsV=kV  UnitsW=MW  buscounter=0  FunctionMessages=off  echomessages=off  EnableUseOfTLC=off  CurrentSourceSwitches=off  DisableSnubberDevices=off  DisableRonSwitches=off  DisableVfSwitches=off  DisplayEquations=off  AutomaticDiscreteSolvers=off  SolverType=Tustin/Backward Euler (TBE)  Interpol=off  ExternalGateDelay=off  methode=off  Ts=100  x0status=blocks  SPID=on  SwTol=0  HookPort=off  NonlinearTolerance=1e-4  nMaxIteration=100  ContinueOnMaxIteration=off  RestoreLinks=warning  ResistiveCurrentMeasurement=off  Frange=[45:5:55]  Ylog=off  Xlog=on  ShowGrid=off  save=off  variable=ZData  structure=H_Last  ZoomFFT=off  StartTime=8.8  cycles=10  DisplayStyle=1  fundamental=50  FreqAxis=on  MaxFrequency=2050  frequencyindicesteady=1  RmsSteady=1  display=off
  switch on : Step  Time=ZK_Belastung_on  SampleTime=0
  switch on1 : Step  Time=0  Before=1  SampleTime=0
  switch on2 : Step  Time=ZK_Belastung_off  SampleTime=0
  tag scope: In_A=global, In_B=global, In_C=global, In_D=global, In_G=global, In_H=global, Messung_Zwischenkreis=global
  wires:
  Current Measurement2/1 -> [In_B]
  Current Measurement3/1 -> [In_A]
  Current Measurement4/1 -> [In_D]
  [Sollwerte_Shunt_U] -> VSC_Shunt_U/1(Sollwerte_Uabc), Sollwertquelle_Shunt_U/1(Sollwerte_Uabc)
  [Sollwerte_Series_U] -> VSC_Series_U/1(Sollwerte_Uabc), Sollwertquelle_Series_U/1(Sollwerte_Uabc)
  Breaker Series Control/1 -> BreakerCtrlSig_Scope/1, L1 Breaker Series/1, L2 Breaker Series/1, L3 Breaker Series/1
  Breaker Shunt Control/1 -> Three-Phase Breaker Shunt/1, N Breaker Shunt/1
  Zwischenkreis_Shunt/1(U DC Zwischenkreis) -> Manual Switch/1  "U DC Zwischenkreis1"
  Zwischenkreis_Series/1(U DC Zwischenkreis) -> Manual Switch1/1  "U DC Zwischenkreis2"
  Zwischenkreis_Shunt/2(I DC Zwischenkreis out) -> Bus Creator/3  "I DC out1"
  Zwischenkreis_Series/2(I DC Zwischenkreis in) -> Bus Creator/4  "I DC in2"
  Zwischenkreis_Shunt/3(I DC Zwischenkreis in) -> Bus Creator/5  "I DC in1"
  Zwischenkreis_Series/3(I DC Zwischenkreis out) -> Bus Creator/6  "I DC out2"
  Bus Creator/1 -> [Messung_Zwischenkreis]
  VSC_Series_U/1(Gatesignale_(6)) -> VSC_Series_SPWM_Scope/1
  Transformator mit Messung/2(U_W1_W2_W3) -> Strom Spannung Trafowicklungen Primär/1  "U_W1_W2_W3"
  Transformator mit Messung/1(I_W1_W2_W3) -> Strom Spannung Trafowicklungen Primär/2  "I_W1_W2_W3"
  Freilaufdioden/1(Out1) -> FreilaufDioden_Scope/1
  VSC_Shunt_U/1(Gatesignale_(6)) -> VSC_Shunt_SPWM_Scope/1
  switch on/1 -> Add/1
  Add/1 -> Ideal Switch/1
  switch on2/1 -> Add/2
  Current Measurement1/1 -> [In_C]
  Current Measurement/1 -> I_Last_Oberschwingung_Scope/1
  Current Measurement6/1 -> I_Last_Oberschwingung_Scope/2
  Current Measurement7/1 -> I_Last_Oberschwingung_Scope/3
  switch on1/1 -> Three-Phase Breaker/1, Switch_Grundlast_Scope/1
  Manual Switch1/1 -> Bus Creator/2  "U DC Zwischenkreis2"
  Manual Switch/1 -> Bus Creator/1  "U DC Zwischenkreis1"
  Constant/1 -> Manual Switch1/2, Manual Switch/2
  Current Measurement8/1 -> [In_G]
  Current Measurement9/1 -> [In_H]
  Breaker Series Control1/1 -> Three-Phase Breaker Shunt1/1
  connections:
  Current Measurement3/LConn1 -- Subsystem/RConn4 -- Ground2/LConn1
  Position 1/RConn1 -- Leitungsnachbildung RL/LConn1
  Position 1/RConn2 -- Leitungsnachbildung RL/LConn2
  Position 1/RConn3 -- Leitungsnachbildung RL/LConn3
  Grundlast/LConn3 -- Three-Phase Breaker/RConn3
  Grundlast/RConn1 -- Oberschwingung Last/LConn1 -- Flicker Last/LConn1 -- Unsymmetrie Last/LConn1 -- RVC Last/LConn1 -- Current Measurement9/RConn1
  Three-Phase Breaker/LConn2 -- Current Measurement6/RConn1 -- Flicker Last/RConn2 -- Unsymmetrie Last/RConn2 -- Messpunkt H/RConn2 -- RVC Last/RConn2
  Position 2/LConn1 -- Leitungsnachbildung RL/RConn1
  Position 2/LConn2 -- Leitungsnachbildung RL/RConn2
  Position 2/LConn3 -- Leitungsnachbildung RL/RConn3
  Current Measurement2/LConn1 -- Leitungsnachbildung RL/RConn4
  Position 3/LConn3 -- Position 2/RConn3
  N Breaker Shunt/RConn1 -- Current Measurement4/LConn1
  LC Filter Series/LConn4 -- L Filter Series/LConn4 -- LCL Filter Series/LConn4
  Position 3/LConn1 -- Position 2/RConn1
  Current Measurement1/LConn1 -- N Breaker Shunt/LConn1 -- Current Measurement2/RConn1
  L Filter Shunt/RConn2 -- Sollwertquelle_Shunt_U/RConn2 -- VSC_Shunt_U/RConn2 -- LCL Filter Shunt/RConn2 -- LC Filter Shunt/RConn2
  LC Filter Shunt/RConn4 -- L Filter Shunt/RConn4 -- LCL Filter Shunt/RConn4
  L Filter Series/LConn1 -- LC Filter Series/LConn1 -- LCL Filter Series/LConn1 -- Wechselrichter Reihe Strom/ Spannung/RConn1
  LCL Filter Series/LConn2 -- L Filter Series/LConn2 -- LC Filter Series/LConn2 -- Wechselrichter Reihe Strom/ Spannung/RConn2
  LCL Filter Series/LConn3 -- L Filter Series/LConn3 -- LC Filter Series/LConn3 -- Wechselrichter Reihe Strom/ Spannung/RConn3
  Shunt Strom/ Spannung/LConn1 -- Three-Phase Breaker Shunt/RConn1
  Shunt Strom/ Spannung/LConn2 -- Three-Phase Breaker Shunt/RConn2
  Shunt Strom/ Spannung/LConn3 -- Three-Phase Breaker Shunt/RConn3
  Ideal Switch/RConn1 -- Series RLC Branch4/LConn1
  LCL Filter Shunt/RConn1 -- L Filter Shunt/RConn1 -- LC Filter Shunt/RConn1 -- Sollwertquelle_Shunt_U/RConn1 -- VSC_Shunt_U/RConn1
  LCL Filter Shunt/RConn3 -- Sollwertquelle_Shunt_U/RConn3 -- L Filter Shunt/RConn3 -- VSC_Shunt_U/RConn3 -- LC Filter Shunt/RConn3
  Three-Phase Breaker Shunt1/LConn2 -- Freilaufdioden/LConn2
  Three-Phase Breaker Shunt1/LConn1 -- Freilaufdioden/LConn1
  Three-Phase Breaker Shunt1/LConn3 -- Freilaufdioden/LConn3
  Current Measurement/LConn1 -- Oberschwingung Last/RConn1
  Oberschwingung Last/RConn2 -- Current Measurement6/LConn1
  Oberschwingung Last/RConn3 -- Current Measurement7/LConn1
  Flicker Last/RConn1 -- Three-Phase Breaker/LConn1 -- Current Measurement/RConn1 -- Unsymmetrie Last/RConn1 -- Messpunkt H/RConn1 -- RVC Last/RConn1
  Unsymmetrie Last/RConn3 -- Three-Phase Breaker/LConn3 -- Current Measurement7/RConn1 -- Flicker Last/RConn3 -- Messpunkt H/RConn3 -- RVC Last/RConn3
  VSC_Series_U/LConn1 -- Ideal Switch/LConn1 -- Zwischenkreis_Series/RConn1
  Series RLC Branch4/RConn1 -- VSC_Series_U/LConn2 -- Zwischenkreis_Series/RConn2
  Position 3/LConn2 -- Position 2/RConn2
  Transformator mit Messung/RConn2 -- Measurement Transformer/LConn5 -- L3 Breaker Series/RConn1 -- Position 3/RConn3
  VSC_Series_U/RConn2 -- Sollwertquelle_Series_U/RConn2 -- L Filter Series/RConn2 -- LC Filter Series/RConn2 -- LCL Filter Series/RConn2
  VSC_Series_U/RConn1 -- Sollwertquelle_Series_U/RConn1 -- L Filter Series/RConn1 -- LC Filter Series/RConn1 -- LCL Filter Series/RConn1
  L Filter Series/RConn4 -- LCL Filter Series/RConn4 -- LC Filter Series/RConn4
  Zwischenkreis_Shunt/LConn2 -- VSC_Shunt_U/LConn2
  Zwischenkreis_Shunt/LConn1 -- VSC_Shunt_U/LConn1
  Sollwertquelle_Series_U/RConn3 -- L Filter Series/RConn3 -- LC Filter Series/RConn3 -- LCL Filter Series/RConn3 -- VSC_Series_U/RConn3
  Three-Phase Breaker Shunt1/RConn1 -- Transformator mit Messung/LConn1 -- Wechselrichter Reihe Strom/ Spannung/LConn1
  Three-Phase Breaker Shunt1/RConn2 -- Wechselrichter Reihe Strom/ Spannung/LConn2 -- Transformator mit Messung/LConn2
  Three-Phase Breaker Shunt1/RConn3 -- Wechselrichter Reihe Strom/ Spannung/LConn3 -- Transformator mit Messung/LConn3
  Leitungsnachbildung RL1/RConn1 -- Messpunkt H/LConn1
  Leitungsnachbildung RL1/RConn2 -- Messpunkt H/LConn2
  Leitungsnachbildung RL1/RConn3 -- Messpunkt H/LConn3
  Current Measurement3/RConn1 -- Leitungsnachbildung RL/LConn4
  Subsystem/RConn1 -- Position 1/LConn1
  Subsystem/RConn2 -- Position 1/LConn2
  Subsystem/RConn3 -- Position 1/LConn3
  DC_Quelle_Zwischenkreis/RConn1 -- Series RLC Branch3/RConn1
  Series RLC Branch1/LConn1 -- Zwischenkreis_Shunt/RConn2 -- Zwischenkreis_Series/LConn2
  Series RLC Branch3/LConn1 -- Zwischenkreis_Shunt/RConn1 -- Zwischenkreis_Series/LConn1
  DC_Quelle_Zwischenkreis/RConn2 -- Series RLC Branch1/RConn1
  Messpunkt C/RConn1 -- Messpunkt G/LConn1 -- Three-Phase Breaker Shunt/LConn1
  Messpunkt C/RConn3 -- Messpunkt G/LConn3 -- Three-Phase Breaker Shunt/LConn3
  Messpunkt C/LConn1 -- L1 Breaker Series/LConn1 -- Transformator mit Messung/RConn5 -- Measurement Transformer/LConn2
  Three-Phase Breaker Shunt/LConn2 -- Messpunkt C/RConn2 -- Messpunkt G/LConn2
  Messpunkt G/RConn3 -- Leitungsnachbildung RL1/LConn3
  Messpunkt G/RConn2 -- Leitungsnachbildung RL1/LConn2
  Messpunkt G/RConn1 -- Leitungsnachbildung RL1/LConn1
  Leitungsnachbildung RL1/LConn4 -- Current Measurement8/RConn1
  Current Measurement8/LConn1 -- Current Measurement1/RConn1
  Current Measurement9/LConn1 -- Leitungsnachbildung RL1/RConn4
  Grundlast/LConn1 -- Three-Phase Breaker/RConn1
  Grundlast/LConn2 -- Three-Phase Breaker/RConn2
  Shunt Strom/ Spannung/RConn1 -- LCL Filter Shunt/LConn1 -- L Filter Shunt/LConn1 -- LC Filter Shunt/LConn1
  Shunt Strom/ Spannung/RConn2 -- L Filter Shunt/LConn2 -- LC Filter Shunt/LConn2 -- LCL Filter Shunt/LConn2
  Shunt Strom/ Spannung/RConn3 -- L Filter Shunt/LConn3 -- LC Filter Shunt/LConn3 -- LCL Filter Shunt/LConn3
  Current Measurement4/RConn1 -- L Filter Shunt/LConn4 -- LC Filter Shunt/LConn4 -- LCL Filter Shunt/LConn4
  Transformator mit Messung/RConn4 -- L2 Breaker Series/RConn1 -- Position 3/RConn2 -- Measurement Transformer/LConn3
  Messpunkt C/LConn3 -- L3 Breaker Series/LConn1 -- Measurement Transformer/LConn6 -- Transformator mit Messung/RConn1
  L2 Breaker Series/LConn1 -- Messpunkt C/LConn2 -- Transformator mit Messung/RConn3 -- Measurement Transformer/LConn4
  Transformator mit Messung/RConn6 -- Measurement Transformer/LConn1 -- Position 3/RConn1 -- L1 Breaker Series/RConn1

== system UPQC_model/DC_Quelle_Zwischenkreis ==
  DC Voltage Source : powerlib/Electrical Sources/DC Voltage Source  Amplitude=U_Zwischenkreis/2  Measurements=None
  DC Voltage Source1 : powerlib/Electrical Sources/DC Voltage Source  Amplitude=U_Zwischenkreis/2  Measurements=None
  Ground1 : powerlib/Elements/Ground  LConnTagsString=a
  Series RLC Branch : powerlib/Elements/Series RLC Branch  LConnTagsString=__new0  RConnTagsString=__new0  BranchType=R  Resistance=1000000  Inductance=1e-3  SetiL0=off  InitialCurrent=0  Capacitance=1e-6  Setx0=off  InitialVoltage=0  Measurements=None
  DC+ : PMIOPort  Side=Right
  DC- : PMIOPort  Port=2  Side=Right
  connections:
  DC Voltage Source/RConn1 -- DC+/RConn1
  DC Voltage Source1/LConn1 -- DC-/RConn1
  DC Voltage Source1/RConn1 -- Series RLC Branch/RConn1 -- DC Voltage Source/LConn1
  Series RLC Branch/LConn1 -- Ground1/LConn1

== system UPQC_model/Flicker Last ==
  Breaker : powerlib/Elements/Breaker  InitialState=0  SwitchingTimes=Flicker_Schaltzeitpunkte_L1  External=off  BreakerResistance=0.01  SnubberResistance=1e6  SnubberCapacitance=inf  Measurements=None  MoreParameters=on  NoBreakLoop=off
  Breaker1 : powerlib/Elements/Breaker  InitialState=0  SwitchingTimes=Flicker_Schaltzeitpunkte_L3  External=off  BreakerResistance=0.01  SnubberResistance=1e6  SnubberCapacitance=inf  Measurements=None  MoreParameters=on  NoBreakLoop=off
  Breaker6 : powerlib/Elements/Breaker  InitialState=0  SwitchingTimes=Flicker_Schaltzeitpunkte_L2  External=off  BreakerResistance=0.01  SnubberResistance=1e6  SnubberCapacitance=inf  Measurements=None  MoreParameters=on  NoBreakLoop=off
  Parallel RLC Load : powerlib/Elements/Parallel RLC Load  LConnTagsString=a  RConnTagsString=__new0  NominalVoltage=230.9  NominalFrequency=50  ActivePower=Pl_Flicker(1)  InductivePower=Ql_ind_Flicker(1)  CapacitivePower=Ql_kap_Flicker(1)  Setx0=off  InitialVoltage=0  SetiL0=off  InitialCurrent=0  Measurements=None  LoadType=constant Z
      settings: AttributesFormatString=\n  SourceProductBaseCode=PS
  Parallel RLC Load1 : powerlib/Elements/Parallel RLC Load  LConnTagsString=a  RConnTagsString=__new0  NominalVoltage=230.9  NominalFrequency=50  ActivePower=Pl_Flicker(2)  InductivePower=Ql_ind_Flicker(2)  CapacitivePower=Ql_kap_Flicker(2)  Setx0=off  InitialVoltage=0  SetiL0=off  InitialCurrent=0  Measurements=None  LoadType=constant Z
      settings: AttributesFormatString=\n  SourceProductBaseCode=PS
  Parallel RLC Load2 : powerlib/Elements/Parallel RLC Load  LConnTagsString=a  RConnTagsString=__new0  NominalVoltage=230.9  NominalFrequency=50  ActivePower=Pl_Flicker(3)  InductivePower=Ql_ind_Flicker(3)  CapacitivePower=Ql_kap_Flicker(3)  Setx0=off  InitialVoltage=0  SetiL0=off  InitialCurrent=0  Measurements=None  LoadType=constant Z
      settings: AttributesFormatString=\n  SourceProductBaseCode=PS
  N : PMIOPort  Side=Left
  L1 : PMIOPort  Port=2  Side=Right
  L2 : PMIOPort  Port=3  Side=Right
  L3 : PMIOPort  Port=4  Side=Right
  connections:
  Breaker1/LConn1 -- Parallel RLC Load2/RConn1
  L3/RConn1 -- Breaker1/RConn1
  Breaker6/LConn1 -- Parallel RLC Load1/RConn1
  Breaker6/RConn1 -- L2/RConn1
  Parallel RLC Load/RConn1 -- Breaker/LConn1
  Breaker/RConn1 -- L1/RConn1
  Parallel RLC Load/LConn1 -- Parallel RLC Load1/LConn1 -- Parallel RLC Load2/LConn1 -- N/RConn1

== system UPQC_model/Freilaufdioden ==
  Diode{,1..3} (4 alike) : powerlib/Power Electronics/Diode  Ron=0.001  Lon=0  Vf=0.8  IC=0  UseSnubber=0  Rs=500  Cs=250e-9  Measurements=on
  Mux : Mux
  A : PMIOPort  Side=Left
  B : PMIOPort  Port=2  Side=Left
  C : PMIOPort  Port=3  Side=Left
  Out1 : Outport
  wires:
  Diode1/1 -> Mux/2  "BC"
  Diode2/1 -> Mux/4  "BA"
  Mux/1 -> Out1/1
  Diode/1 -> Mux/1  "AB"
  Diode3/1 -> Mux/3  "CB"
  connections:
  Diode/LConn1 -- A/RConn1 -- Diode2/RConn1
  Diode/RConn1 -- Diode2/LConn1 -- Diode3/RConn1 -- B/RConn1 -- Diode1/LConn1
  Diode1/RConn1 -- Diode3/LConn1 -- C/RConn1
